simulink model "observerStateFeedback"  (R2024b)
settings: Solver=VariableStepAuto  StartTime=0.0  StopTime=1  RelTol=1e-3
undefined symbols (not defined in the file): A, B, C, K, L, r, x_0
settings Model: Creator=Longbin  LastModifiedBy=Longbin

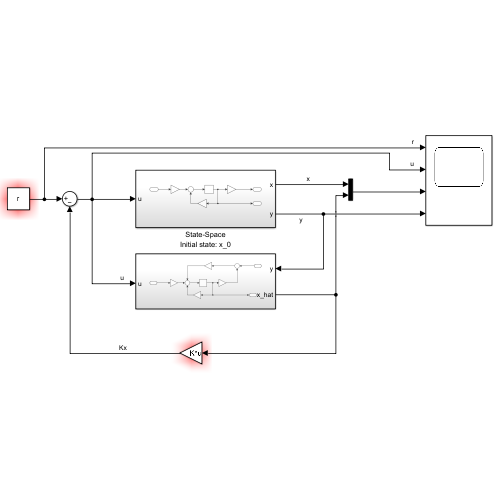
[thumbnail: Simulink's stored preview of the top-level diagram]
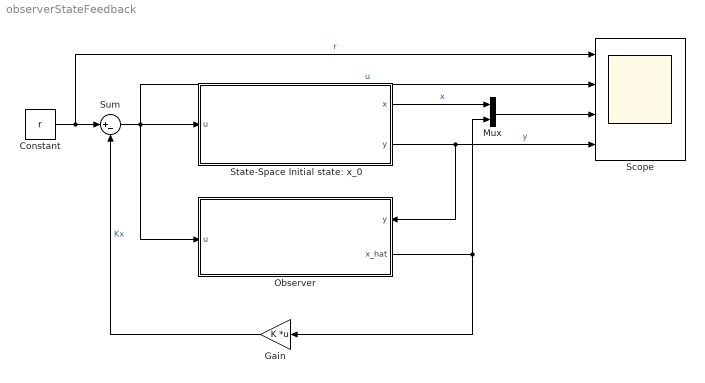
== system observerStateFeedback ==
  Constant : Constant  Value=r
  Gain : Gain  Gain=K  Multiplication=Matrix(K*u)
  Mux : Mux  Inputs=2
  Observer : Subsystem
      settings: PortSchema="{\"entries\":[{\"content\":{\"sides\":[{\"content\":{\"connectorIds\":[\"In1\"]},\"type\":\"ConnectorPlacement.EquallySpacedRectSide\",\"uuid\":\"545bea58-88b4-4d16-be1c-dd1ec5015899\"},{\"content\":{\"connectorIds\":[\"In2\",\"Out1\"],\"side\":\"RIGHT\"},\"type\":\"ConnectorPlacement.EquallySpacedRectSide\",\"uuid\":\"d40df04c-a1a7-496b-9f64-1f7964fa4ba0\"},{\"content\":{\"side\":\"TOP\"},\"type\":\"ConnectorPlacement.EquallySpacedRectSide\",\"uuid\":\"5ee1fb98-44ef-48cb-a735-1a4d6f7c2527\"}]},\"type\":\"ConnectorPlacement.EquallySpacedConnector\",\"uuid\":\"a8527127-b43c-4135-914b-42c25a844472\"}],\"packageUris\":[\"http://schema.mathworks.com/mf0/Connector/R2020b\"],\"version\":\"1.0\"}"
  Scope : Scope  NumInputPorts=4
  State-Space Initial state: x_0 : Subsystem
  Sum : Sum  Inputs=|+-
  wires:
  Gain/1 -> Sum/2  "Kx"
  Constant/1 -> Scope/1, Sum/1  "r"
  Sum/1 -> Scope/2, State-Space Initial state: x_0/1(u), Observer/1(u)  "u"
  Mux/1 -> Scope/3
  State-Space Initial state: x_0/2(y) -> Observer/2(y), Scope/4  "y"
  State-Space Initial state: x_0/1(x) -> Mux/1  "x"
  Observer/1(x_hat) -> Gain/1, Mux/2

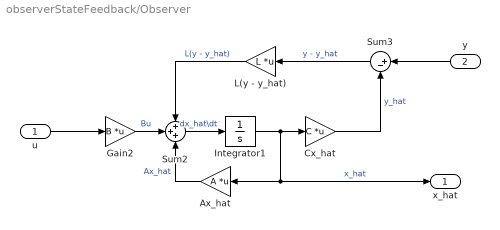
== system observerStateFeedback/Observer ==
  u : Inport
  y : Inport  Port=2
  Ax_hat : Gain  Gain=A  Multiplication=Matrix(K*u)
  Cx_hat : Gain  Gain=C  Multiplication=Matrix(K*u)
  Gain2 : Gain  Gain=B  Multiplication=Matrix(K*u)
  Integrator1 : Integrator
  L(y - y_hat) : Gain  Gain=L  Multiplication=Matrix(K*u)
  Sum2 : Sum  Inputs=+++
  Sum3 : Sum  Inputs=|+-
  x_hat : Outport
  wires:
  Sum3/1 -> L(y - y_hat)/1  "y - y_hat"
  Gain2/1 -> Sum2/2  "Bu"
  Cx_hat/1 -> Sum3/2  "y_hat"
  L(y - y_hat)/1 -> Sum2/1  "L(y - y_hat)"
  Sum2/1 -> Integrator1/1  "dx_hat\\dt"
  Integrator1/1 -> Ax_hat/1, x_hat/1, Cx_hat/1  "x_hat"
  Ax_hat/1 -> Sum2/3  "Ax_hat"
  y/1 -> Sum3/1
  u/1 -> Gain2/1

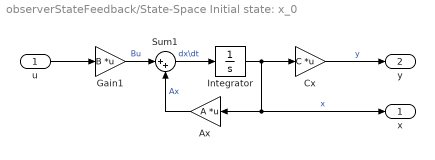
== system observerStateFeedback/State-Space Initial state: x_0 ==
  u : Inport
  Ax : Gain  Gain=A  Multiplication=Matrix(K*u)
  Cx : Gain  Gain=C  Multiplication=Matrix(K*u)
  Gain1 : Gain  Gain=B  Multiplication=Matrix(K*u)
  Integrator : Integrator  InitialCondition=x_0
  Sum1 : Sum  Inputs=|++
  x : Outport
  y : Outport  Port=2
  wires:
  Integrator/1 -> Cx/1, x/1, Ax/1  "x"
  Gain1/1 -> Sum1/1  "Bu"
  Ax/1 -> Sum1/2  "Ax"
  Cx/1 -> y/1  "y"
  Sum1/1 -> Integrator/1  "dx\\dt"
  u/1 -> Gain1/1
